simulink subsystem "myTHD_fixed"  (R2024a)
settings: Solver=VariableStepAuto  StartTime=0.0  StopTime=10.0  RelTol=1e-3
values from neighbouring files (symbols this model uses):
  a = 1/data(end, 1)    [csv_analize.m]
  b = 1/data(2, 1)    [csv_analize.m]
undefined symbols (not defined in the file or in its folder): BUFFER_LEN, c, MAIN_FREQ_INDEX, SAMPLING_FREQ
libraries: hdlsllib x4, dspsigops x3, embmathops x2, embreciprocals x1, simulink_extras x1
settings Model: Creator=Jan Rosa  LastModifiedBy=Jan Rosa

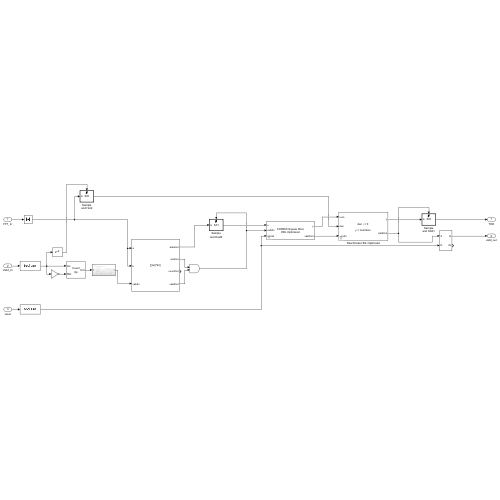
[thumbnail: Simulink's stored preview of the top-level diagram]
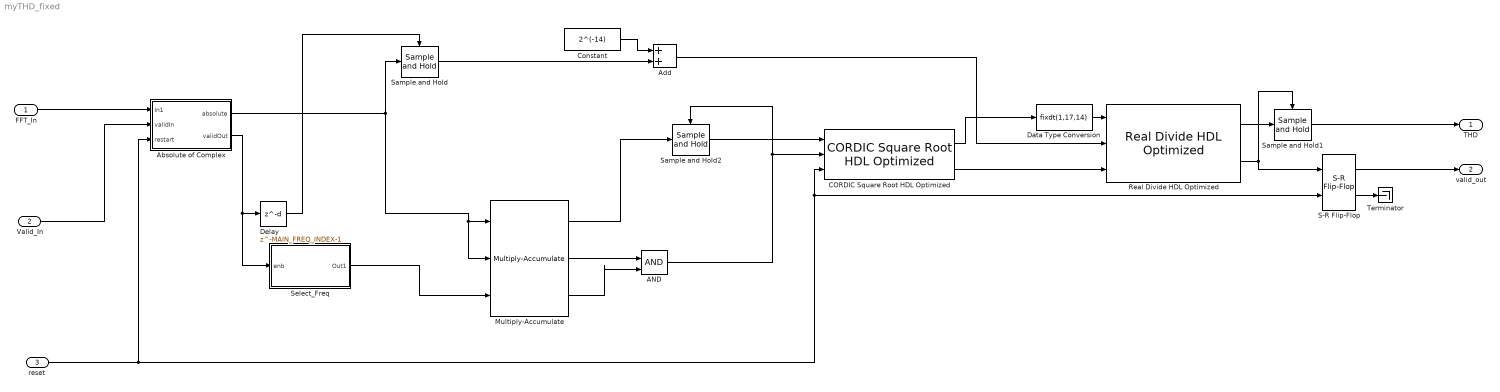
== system myTHD_fixed ==
  FFT_In : Inport
  Valid_In : Inport  Port=2
  reset : Inport  Port=3
  AND : Logic  IconShape=distinctive  AllPortsSameDT=off  OutDataTypeStr=boolean
  Absolute of Complex : Subsystem  TreatAsAtomicUnit=on
  Add : Sum
  CORDIC Square Root HDL Optimized : embmathops/CORDIC Square Root HDL Optimized  autoMaximumShiftVal=on  maximumShiftValue=10  nIterPerReg=1
      settings: LibrarySourceBlock=embeddedMatrixLib/Math Operations/CORDIC Square Root HDL Optimized
  Constant : Constant  Value=2^(-14)  OutDataTypeStr=fixdt(1,16,14)  SampleTime=1/SAMPLING_FREQ
  Data Type Conversion : DataTypeConversion  OutDataTypeStr=fixdt(1,17,14)  SaturateOnIntegerOverflow=off  RndMeth=Floor
  Delay : Delay  DelayLength=MAIN_FREQ_INDEX-1
  Multiply-Accumulate : hdlsllib/HDL Operations/Multiply-Accumulate  opMode=Streaming - using Number of Samples  initValueSetting=Dialog  initValue=0  initValueSetting2=Dialog  initValue2=0  initValueSetting3=Dialog  initValue3=0  num_samples=(BUFFER_LEN/2 - MAIN_FREQ_INDEX)  RndMeth2=Floor  RndMeth3=Floor  datatype2=Inherit: Inherit via back propagation  datatype3=fixdt(1,22,20)  validOut=on  endInandOut=on  startOut=on  countOut=off  dim=-1  DoSatur=off  parallel=off
  Real Divide HDL Optimized : embreciprocals/Real Divide HDL Optimized  OutputType=fixdt(1,18,10)
      settings: LibrarySourceBlock=embeddedMatrixLib/Math Operations/Real Divide HDL Optimized
  S-R Flip-Flop : simulink_extras/Flip Flops/S-R Flip-Flop  initial_condition=0
  Sample and Hold : dspsigops/Sample and Hold  trig=Rising edge  initCond=0  latchinput=off
  Sample and Hold1 : dspsigops/Sample and Hold  trig=Rising edge  initCond=0  latchinput=off
  Sample and Hold2 : dspsigops/Sample and Hold  trig=Rising edge  initCond=0  latchinput=off
  Select_Freq : Subsystem  TreatAsAtomicUnit=on
  Terminator : Terminator
  THD : Outport
  valid_out : Outport  Port=2
  wires:
  CORDIC Square Root HDL Optimized/2 -> Real Divide HDL Optimized/3
  Real Divide HDL Optimized/1 -> Sample and Hold1/1
  S-R Flip-Flop/2 -> Terminator/1
  Data Type Conversion/1 -> Real Divide HDL Optimized/1
  S-R Flip-Flop/1 -> valid_out/1
  CORDIC Square Root HDL Optimized/1 -> Data Type Conversion/1
  Real Divide HDL Optimized/2 -> Sample and Hold1/Trigger, S-R Flip-Flop/1
  Sample and Hold1/1 -> THD/1
  Multiply-Accumulate/1 -> Sample and Hold2/1
  Add/1 -> Real Divide HDL Optimized/2
  AND/1 -> Sample and Hold2/Trigger, CORDIC Square Root HDL Optimized/2
  Sample and Hold2/1 -> CORDIC Square Root HDL Optimized/1
  Constant/1 -> Add/1
  Sample and Hold/1 -> Add/2
  Absolute of Complex/2(validOut) -> Delay/1, Select_Freq/1(enb)
  reset/1 -> CORDIC Square Root HDL Optimized/3, S-R Flip-Flop/2, Absolute of Complex/3(restart)
  Absolute of Complex/1(absolute) -> Sample and Hold/1, Multiply-Accumulate/1, Multiply-Accumulate/2
  FFT_In/1 -> Absolute of Complex/1(In1)
  Valid_In/1 -> Absolute of Complex/2(validIn)
  Delay/1 -> Sample and Hold/Trigger
  Multiply-Accumulate/2 -> AND/1
  Multiply-Accumulate/3 -> AND/2
  Select_Freq/1(Out1) -> Multiply-Accumulate/3

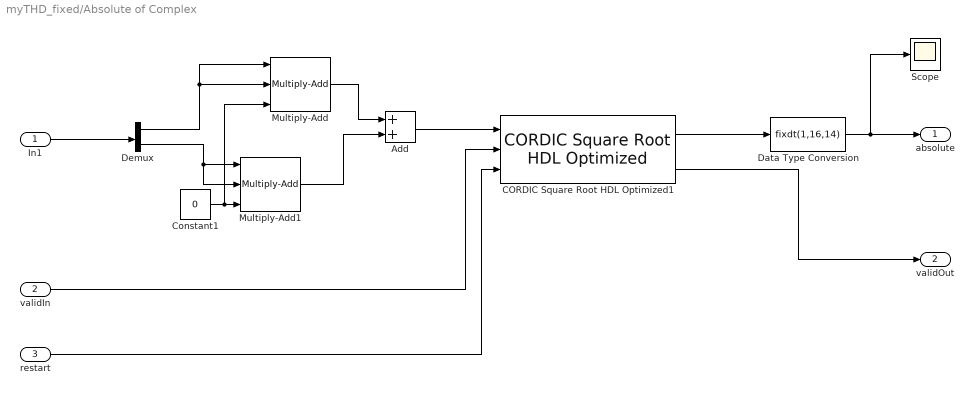
== system myTHD_fixed/Absolute of Complex ==
  In1 : Inport
  validIn : Inport  Port=2
  restart : Inport  Port=3
  Add : Sum
  CORDIC Square Root HDL Optimized1 : embmathops/CORDIC Square Root HDL Optimized  autoMaximumShiftVal=on  maximumShiftValue=10  nIterPerReg=1
      settings: LibrarySourceBlock=embeddedMatrixLib/Math Operations/CORDIC Square Root HDL Optimized
  Constant1 : Constant  Value=0  OutDataTypeStr=fixdt(1,12,11)  SampleTime=1/SAMPLING_FREQ
  Data Type Conversion : DataTypeConversion  OutDataTypeStr=fixdt(1,16,14)  SaturateOnIntegerOverflow=off  RndMeth=Floor
  Demux : Demux  Outputs=2
  Multiply-Add : hdlsllib/HDL Operations/Multiply-Add  Function=c+(a.*b)  datatype=fixdt(1,23,22)  DoSatur=off  FMA=off
  Multiply-Add1 : hdlsllib/HDL Operations/Multiply-Add  Function=c+(a.*b)  datatype=fixdt(1,23,22)  DoSatur=off  FMA=off
  Scope : Scope
  absolute : Outport
  validOut : Outport  Port=2
  wires:
  Data Type Conversion/1 -> absolute/1, Scope/1
  CORDIC Square Root HDL Optimized1/2 -> validOut/1
  validIn/1 -> CORDIC Square Root HDL Optimized1/2
  CORDIC Square Root HDL Optimized1/1 -> Data Type Conversion/1
  In1/1 -> Demux/1
  Add/1 -> CORDIC Square Root HDL Optimized1/1
  Demux/1 -> Multiply-Add/2, Multiply-Add/1
  Demux/2 -> Multiply-Add1/1, Multiply-Add1/2
  Constant1/1 -> Multiply-Add1/3, Multiply-Add/3
  restart/1 -> CORDIC Square Root HDL Optimized1/3
  Multiply-Add/1 -> Add/1
  Multiply-Add1/1 -> Add/2

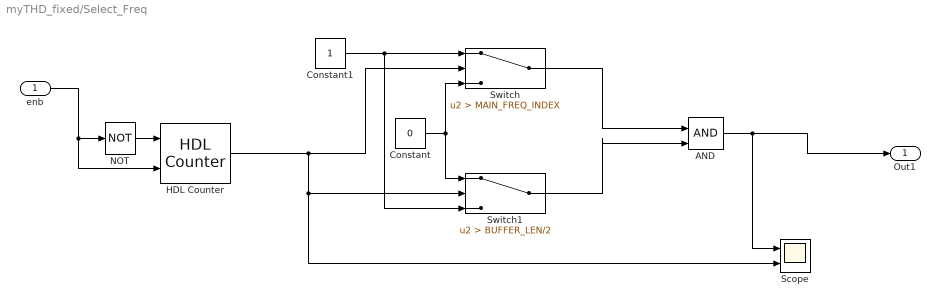
== system myTHD_fixed/Select_Freq ==
  enb : Inport  OutDataTypeStr=boolean
  AND : Logic  IconShape=distinctive  AllPortsSameDT=off  OutDataTypeStr=boolean
  Constant : Constant  Value=0  OutDataTypeStr=boolean  SampleTime=1/SAMPLING_FREQ
  Constant1 : Constant  OutDataTypeStr=boolean  SampleTime=1/SAMPLING_FREQ
  HDL Counter : hdlsllib/Sources/HDL Counter  CountType=Count limited  CountInit=0  CountStep=1  CountMax=BUFFER_LEN  CountFromType=Initial value  CountFrom=0  CountResetPort=on  CountLoadPort=off  CountEnbPort=on  CountDirPort=off  CountHitOutputPort=off  CountDataType=Unsigned  CountWordLen=12  CountFracLen=0  CountSampTime=1
  NOT : Logic  Operator=NOT  IconShape=distinctive  AllPortsSameDT=off  OutDataTypeStr=boolean
  Scope : Scope  NumInputPorts=2
  Switch : Switch  Criteria=u2 > Threshold  Threshold=MAIN_FREQ_INDEX  SaturateOnIntegerOverflow=off  InputSameDT=off
  Switch1 : Switch  Criteria=u2 > Threshold  Threshold=BUFFER_LEN/2  SaturateOnIntegerOverflow=off  InputSameDT=off
  Out1 : Outport  OutDataTypeStr=boolean
  wires:
  Switch/1 -> AND/1
  Switch1/1 -> AND/2
  Constant1/1 -> Switch1/3, Switch/1
  Constant/1 -> Switch/3, Switch1/1
  HDL Counter/1 -> Switch/2, Scope/2, Switch1/2
  AND/1 -> Scope/1, Out1/1
  NOT/1 -> HDL Counter/1
  enb/1 -> NOT/1, HDL Counter/2
